simulink model "untitled1"  (R2018a)
settings: Solver=VariableStepAuto  StartTime=0.0  StopTime=10.0  RelTol=1e-3
settings Model: Creator=86188  LastModifiedBy=86188

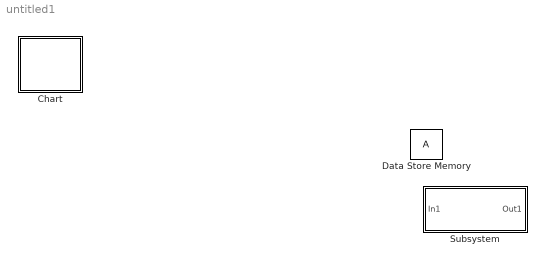
== system untitled1 ==
  Chart : Stateflow chart  TreatAsAtomicUnit=on
  Data Store Memory : DataStoreMemory  ReadBeforeWriteMsg=warning  WriteAfterWriteMsg=warning  WriteAfterReadMsg=warning  ShowAdditionalParam=off
  Subsystem : Subsystem

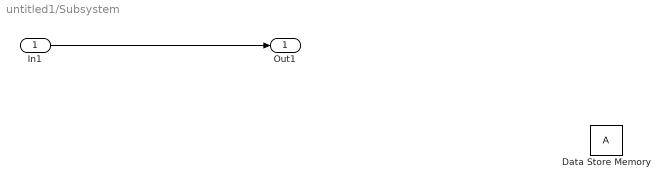
== system untitled1/Subsystem ==
  In1 : Inport
  Data Store Memory : DataStoreMemory  ReadBeforeWriteMsg=warning  WriteAfterWriteMsg=warning  WriteAfterReadMsg=warning  ShowAdditionalParam=off
  Out1 : Outport
  wires:
  In1/1 -> Out1/1

== stateflow chart untitled1/Chart ==
  state count1 = set_final_Flag(wid,count) [function]
    (junction 17) -> (junction 9) [order 2] : {buffer_heartbeat(1)=SET;count1 = count + 1}
    (junction 9) -> (junction 5)
    (default) -> (junction 17)
    (junction 17) -> (junction 16) [order 1] : [count==3]
    (junction 18) -> (junction 9)
    (junction 16) -> (junction 18) : {buffer_heartbeat(1)=NO_SET;count1=0}
  (default) -> (junction 21) : {count3 = set_final_Flag(1,0)}
  data: wid function_input; count function_input; count1 function_output; count3 local =0
